simulink model "Open_loop_sailboat"  (R2017a)
settings: Solver=VariableStepAuto  StartTime=0.0  StopTime=10.0  RelTol=1e-3
PreLoadFcn:
  | load('Sailboat_Constants_1.mat')
libraries: simulink x1
settings Model: Creator=jorda  LastModifiedBy=shim09

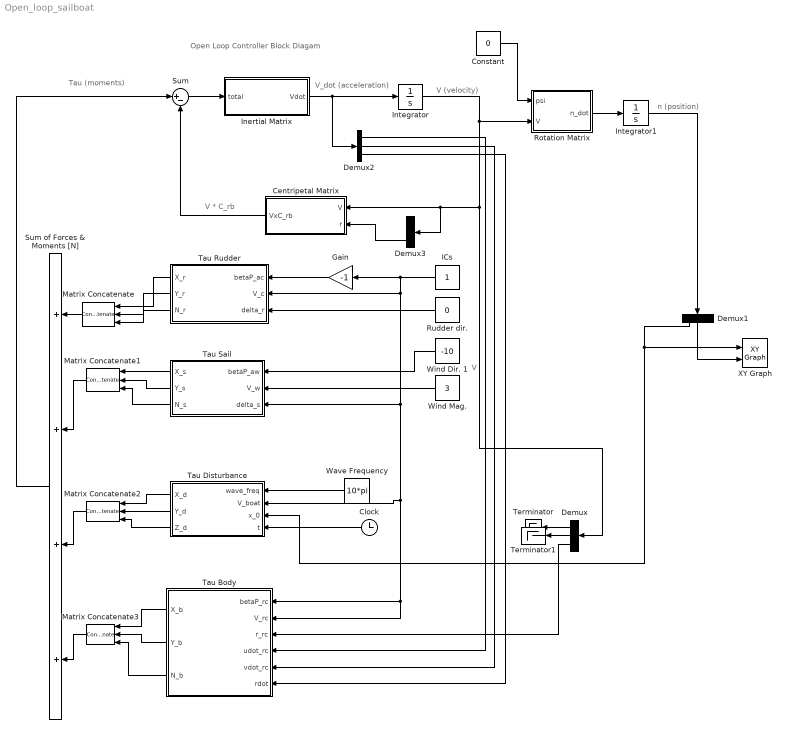
== system Open_loop_sailboat ==
  note: V * C_rb
  note: V
  note: Tau (moments)
  note: V_dot (acceleration)
  note: n (position)
  note: V (velocity)
  note: Open Loop Controller Block Diagam
  "Centripetal Matrix " : MATLAB Function  TreatAsAtomicUnit=on
  Clock : Clock
  Constant : Constant  Value=0
  Demux{,1..3} (4 alike) : Demux  Outputs=3
  Gain : Gain  Gain=-1
  ICs : Constant
  Inertial Matrix : MATLAB Function  TreatAsAtomicUnit=on
  Integrator : Integrator
  Integrator1 : Integrator
  Matrix Concatenate{,1..3} (4 alike) : Concatenate  NumInputs=3  Mode=Multidimensional array
  Rotation Matrix : MATLAB Function  TreatAsAtomicUnit=on
  Rudder dir. : Constant  Value=0
  Sum : Sum  Inputs=|+-
  "Sum of Forces & Moments [N] " : Sum  Inputs=++++
  Tau Body : MATLAB Function  TreatAsAtomicUnit=on
  Tau Disturbance : MATLAB Function  TreatAsAtomicUnit=on
  Tau Rudder : MATLAB Function  TreatAsAtomicUnit=on
  Tau Sail : MATLAB Function  TreatAsAtomicUnit=on
  Terminator : Terminator
  Terminator1 : Terminator
  Wave Frequency : Constant  Value=10*pi
  Wind Dir. 1 : Constant  Value=-10
  "Wind Mag. " : Constant  Value=3
  XY Graph : simulink/Sinks/XY Graph  xmin=-1  xmax=1  ymin=-1  ymax=1  st=-1
  wires:
  Sum/1 -> Inertial Matrix/1(total)
  "Centripetal Matrix "/1(VxC_rb) -> Sum/2
  "Sum of Forces & Moments [N] "/1 -> Sum/1
  Rotation Matrix/1(n_dot) -> Integrator1/1
  Integrator1/1 -> Demux1/1
  Tau Rudder/1(X_r) -> Matrix Concatenate/1
  Tau Rudder/2(Y_r) -> Matrix Concatenate/2
  Tau Rudder/3(N_r) -> Matrix Concatenate/3
  Tau Sail/2(Y_s) -> Matrix Concatenate1/2
  Tau Sail/1(X_s) -> Matrix Concatenate1/1
  Tau Sail/3(N_s) -> Matrix Concatenate1/3
  Matrix Concatenate/1 -> "Sum of Forces & Moments [N] "/1
  Matrix Concatenate1/1 -> "Sum of Forces & Moments [N] "/2
  Tau Disturbance/1(X_d) -> Matrix Concatenate2/1
  Tau Disturbance/2(Y_d) -> Matrix Concatenate2/2
  Tau Disturbance/3(Z_d) -> Matrix Concatenate2/3
  Matrix Concatenate2/1 -> "Sum of Forces & Moments [N] "/3
  Tau Body/1(X_b) -> Matrix Concatenate3/1
  Tau Body/2(Y_b) -> Matrix Concatenate3/2
  Tau Body/3(N_b) -> Matrix Concatenate3/3
  Matrix Concatenate3/1 -> "Sum of Forces & Moments [N] "/4
  Inertial Matrix/1(Vdot) -> Demux2/1, Integrator/1
  Clock/1 -> Tau Disturbance/4(t)
  Integrator/1 -> Demux/1, Demux3/1, "Centripetal Matrix "/1(V), Rotation Matrix/2(V)
  Demux1/1 -> XY Graph/1, Tau Disturbance/3(x_0)
  Gain/1 -> Tau Rudder/1(betaP_ac)
  ICs/1 -> Tau Disturbance/2(V_boat), Tau Body/2(V_rc), Tau Body/1(betaP_rc), Tau Sail/3(delta_s), Tau Rudder/2(V_c), Gain/1
  Demux/3 -> Tau Body/3(r_rc)
  Demux2/1 -> Tau Body/4(udot_rc)
  Demux2/2 -> Tau Body/5(vdot_rc)
  Demux2/3 -> Tau Body/6(rdot)
  Wave Frequency/1 -> Tau Disturbance/1(wave_freq)
  Demux3/3 -> "Centripetal Matrix "/2(r)
  Demux/1 -> Terminator/1
  Demux/2 -> Terminator1/1
  Constant/1 -> Rotation Matrix/1(psi)
  "Wind Mag. "/1 -> Tau Sail/2(V_w)
  Wind Dir. 1/1 -> Tau Sail/1(betaP_aw)
  Rudder dir./1 -> Tau Rudder/3(delta_r)
  Demux1/2 -> XY Graph/2

== matlab function Open_loop_sailboat/Tau Sail ==
  data: betaP_aw input; X_s output; V_w input; Y_s output; N_s output; delta_s input
% Control Surface Force: Sail 
function [X_s,  Y_s,  N_s] = tauSail(betaP_aw, V_w, delta_s)
% Equations for tauSail, control surface force of the sail
% betaP_aw [deg]: direction of the apparent wind velocity, measured clockwise
% from the positive x-axis of the body
% V_w [m/s]: magnitude of the apparent wind velocity 
% delta_s [deg]: angle of the sail

% constants 
C_ls = 1;
rho_w = 1.2250;
S_s = 0.3942;
C_d = 0.75;
b_s = 0.6366;

% based on Equation 5.5: Equations for Lift & Drag 
L_s = C_ls*0.5*rho_w*(V_w^2)*S_s;
D_s = C_d*0.5*rho_w*(V_w^2)*S_s;

% based on Table 5.2: Direction of the Lift force in the Sail 
% if (betaP_aw >= delta_s ) && ((delta_s + 90) >= betaP_aw)
betaPl_aw = betaP_aw + 90/2;
% elseif (betaP_aw >= delta_s + 90) && ((delta_s + 2*90) >= betaP_aw)
%     betaPl_aw = betaP_aw - 90/2;
% end

% based on Equation 5.11
X_s = abs(D_s)*cosd(betaP_aw) + abs(L_s)*cosd(betaPl_aw);
Y_s = abs(D_s)*sind(betaP_aw) + abs(L_s)*sind(betaPl_aw);
N_s = (b_s/4)*Y_s;
end

== matlab function Open_loop_sailboat/Tau Rudder ==
  data: betaP_ac input; X_r output; Y_r output; N_r output; V_c input; delta_r input
% Control Surface Force: Rudder
function [X_r, Y_r, N_r] = tauRudder(betaP_ac, V_c, delta_r)
% Equations for tauRudder, control surface force of the rudder 
% betaP_ac [deg]: direction of the apparent water velocity, measured clockwise
% from the positive x-axis of the body (opposite of boat velocity) 
% V_c [m/s]: magnitude of the apparent water velocity (same as boat
% velocity)
% delta_r [deg]: angle of the rudder 

% constants
C_lr = 1.25;
rho_c = 1000;
S_r = 0.0092;
C_d = 0.75;
b_r = 0.0635;

% based on Equation 5.5: Equations for Lift & Drag 
L_r = C_lr*0.5*rho_c*(V_c^2)*S_r;
D_r = C_d*0.5*rho_c*(V_c^2)*S_r;

% based on Table 5.1: Direction of the Lift force in the rudder
% if (betaP_ac >= delta_r) && ((delta_r + 90) >= betaP_ac)
betaPl_ac = betaP_ac + 90/2;
% elseif (betaP_ac >= delta_r + 90) && ((delta_r + 2*90) >= betaP_ac)
%     betaPl_ac = betaP_ac - 90/2;
% end 

% based on Equation 5.9
X_r = - abs(D_r)*cosd(betaP_ac) + abs(L_r)*cosd(betaPl_ac);
Y_r = abs(D_r)*sind(betaP_ac) + abs(L_r)*sind(betaPl_ac);
N_r = (b_r/4)*Y_r;
end

== matlab function Open_loop_sailboat/Tau Body ==
  data: betaP_rc input; X_b output; Y_b output; N_b output; V_rc input; r_rc input; udot_rc input; vdot_rc input; rdot input
% Body Forces: Rigid Body, Added Mass, and Damping 
function [X_b, Y_b, N_b] = tauBody(betaP_rc, V_rc, r_rc, udot_rc, vdot_rc, rdot)
% Equations for the hydrodynamic body forces on the hull due to the rigid
% body, the added mass, and damping 
% betaP_rc [deg]: direction of the relative sailboat velocity to the current
% (current assumed to have a negligible velocity) 
% V_rc [m/s]: magnitude of the relative sailboat velocity
% r_rc [rad/s]: yaw rate of the sailboat in the z-direction
% udot_rc [m/s^2]: magnitude of the sailboat acceleration in the x-direction
% vdot_rc [m/s^2]: magnitude of the sailboat acceleration in the y-direction
% rdot [rad/s^2]: yaw acceleration of the sailboat in the z-direction

% table 5.3 and other constants for rigid body 
rho_c = 1000;
A_ut = 0.1064;
XP_uu = -0.12;
XP_vv = -0.0890;
XP_ur = 0.0700; 
XP_rr = 0.0110;
XP_vr = 0.0500;
A_ul = 0.3060;
L = 1.0541;
YP_v = -0.244;
YP_vv = -0.9;
YP_r = 0.0790; 
YP_vr = -0.25;
YP_rr = -0.0870;  
NP_v = -0.2;
NP_r = -0.044; 
NP_vrr = 0.07; 
NP_vvr = -0.6;
NP_rr = -0.06; 
% table 5.5 constants for added mass 
X_udot = 0.2310; 
Y_vdot = 9.95;
N_rdot = 8.1; 
% table 5.6 constants for damping forces
X_u = -4.05;
Y_v = 50.8;
Y_r = 1.83;
N_v = -12.5; 
N_r = 2.31; 

% based on Table 5.4 and Equation 5.15: Dimensionless velocities 
uP_rc = cosd(betaP_rc);
vP_rc = sind(betaP_rc);
rP_rc = r_rc*L/V_rc;

% based on Equation 5.14: Equations for the rigid body forces (A_ut & A_ul
% TBD)
X_rb = 0.5*rho_c*A_ut*V_rc^2*(XP_uu*uP_rc^2 + XP_vv*vP_rc^2 + XP_ur*uP_rc*rP_rc + XP_vr*vP_rc*rP_rc + XP_rr*rP_rc^2);
Y_rb = 0.5*rho_c*A_ul*V_rc^2*(YP_v*vP_rc + YP_vv*vP_rc*abs(vP_rc) + YP_r*rP_rc + YP_vr*vP_rc*rP_rc + YP_rr*rP_rc*abs(rP_rc));
N_rb = 0.5*rho_c*A_ul*L^3*V_rc^2*(NP_v*vP_rc + NP_r*rP_rc + NP_vrr*vP_rc*rP_rc^2 + NP_vvr*vP_rc^2*rP_rc + NP_rr*rP_rc*abs(rP_rc));

% based on Equation 5.15: Components of sailboat velocity
u = V_rc*cosd(betaP_rc);       % u_rc = u
v = V_rc*cosd(betaP_rc);       % v_rc = v     
r = r_rc; 

% based on Equation 5.26: Equations for the added mass forces
X_a = X_udot*udot_rc - Y_vdot*v*r; 
Y_a = Y_vdot*vdot_rc + X_udot*u*r;
N_a = N_rdot*rdot + Y_vdot*v*u - X_udot*u*v;

% based on Equation 5.30 and Equation 5.33: Equations for the damping forces
X_da = -X_u*u;
Y_da = -Y_v*v - Y_r*r;
N_da = -N_v*v - N_r *r;

% total amount of forces in X , Y & N in Tau Body 
X_b = X_rb + X_a + X_da;
Y_b = Y_rb + Y_a + Y_da;
N_b = N_rb + N_a + N_da;
end

== matlab function Open_loop_sailboat/Tau Disturbance ==
  data: wave_freq input; X_d output; Y_d output; Z_d output; V_boat input; x_0 input; t input
% Calculations for the disturbance forces for the sailboat simulation.
% Utilizes parameters from the physical boat (beam, length, draft),
% parameters of the fluid (density), and models waves as a sinusoid whose 
% frequency is a function of the velocity of the waves as well as the
% boat velocity. 
%
% Inputs: wave frequency (wave_freq), boat speed (V_boat), wave height (h)
% Outputs: resultant forces and moments component-wise (X_d, Y_d, Z_d)
%
% Assumptions: typical "wave_freq" of lake is 2*pi*(vel/wavelength) = 10*pi,
% wave ht. 1/4m, 
%
% Next: update chi (wave incidence), link time dependent variables to
% Simulink 
%
% Bryan Zhao - 4/6/18

function [X_d, Y_d, Z_d] = tauDisturb(wave_freq, V_boat, x_0, t)


% define constants
T = 0.4064; % draft of boat [m]
L = 1.0541; % length [m]
rho = 1000; % density of water [kg/m^3]
B = 0.3333; % beam of boat [m]
g = 9.81; % std. gravity [m/s^2]
beta_c = 0; % rel. angle between heading and current [deg]
chi = 0; % wave incidence? need to redefine [deg]
h = 1/4; % wave height [m]

% dependencies
k = (4 * pi^2 * wave_freq^2)/ g; % wave number
enc_freq = wave_freq - k*V_boat*cos(chi); % encounter freq.

% wave profile
s = -k*h/2 * sin(k*x_0 - enc_freq*t); % wave slope
eta = (h/2) * cos(k*x_0 - enc_freq*t); % wave profile

X_d = rho * g * B * L * T * cos(beta_c) * s; % X component of tau_disturb
Y_d = -rho * g * B * L * T * sin(beta_c) * s;
Z_d = (1/24) * rho * g * B * L * (L^2 - B^2) * T * k^2 * sin(2*beta_c) * eta;

end

% end of function

== matlab function Open_loop_sailboat/Inertial Matrix ==
  data: total input; Vdot output
function Vdot = M_rb(total)
% Function: The inertial matrix function takes inputs
% 1. forces & moments 2. V*C_rb
% and multiplies the inputs by the inverse of M

% constants 
m_ship = 4;
I_z = 0.09; 

M = [m_ship, 0, 0; 0, m_ship, 0; 0, 0, I_z]; % Inertial Matrix
invM = inv(M);
Vdot = invM*total; % outputs results in V_dot

% JL 4/6/18
% edited JL 4/10/18

== matlab function Open_loop_sailboat/Rotation Matrix ==
  data: psi input; n_dot output; V input
function n_dot = J(psi,V)


R = [ cosd(psi), -sind(psi), 0; sind(psi), cosd(psi),0; 0, 0,1];

n_dot = R*V;

== matlab function Open_loop_sailboat/Centripetal Matrix  ==
  data: V input; VxC_rb output; r input
function VxC_rb = C_rb(V,r)
% function that contains the Centripetal Matrix
% inputs: V (velocity of sailboat)
% outputs: V*C_rb 

%constants 
m_ship = 4; % kg, mass of ship 



C_rb = [ 0, -m_ship*r, 0; m_ship*r, 0, 0; 0,0,0];
VxC_rb = C_rb*V;

end
